simulink model "sinVelToLeader"  (R2016a)
settings: Solver=FixedStepAuto  StartTime=0.0  StopTime=inf  RelTol=1e-3
undefined symbols (not defined in the file or in its folder): Angular, Linear
libraries: robotlib x2
settings Model: Creator=ece446  LastModifiedBy=ece446
settings OptimizationCC: OptimizeModelRefInitCode=on  LifeSpan=Inf  MaxStackSize=64
settings HardwareCC: ProdBitPerPointer=32  ProdLargestAtomicFloat=None  ProdIntDivRoundTo=Undefined  ProdEndianess=Unspecified  ProdWordSize=32  ProdHWDeviceType=Generic->Unspecified (assume 32-bit Generic)  UseEmbeddedCoderFeatures=off
settings RTWCC: SystemTargetFile=ert.tlc  HardwareBoard=Robot Operating System (ROS)  TemplateMakefile=ert_default_tmf  GenerateReport=on  Toolchain=Catkin  IncludeHyperlinkInReport=on  LaunchReport=on  TargetLang=C++  GenerateTraceInfo=on  GenerateTraceReport=on  GenerateTraceReportSl=on  GenerateTraceReportSf=on  GenerateTraceReportEml=on
settings CodeAppCC: ForceParamTrailComments=on  IgnoreCustomStorageClasses=off  OperatorAnnotations=on  SimulinkDataObjDesc=on  SFDataObjDesc=on  MATLABFcnDesc=on  InsertBlockDesc=on  MATLABSourceComments=on
settings ERTTargetCC: SupportNonInlinedSFcns=on

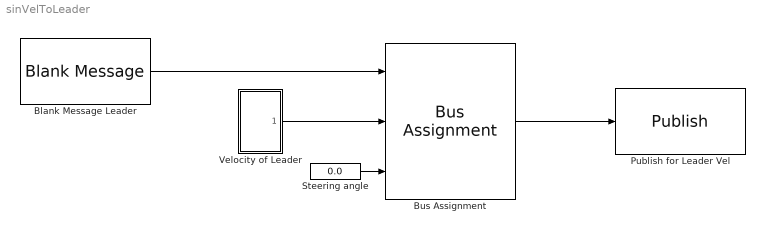
== system sinVelToLeader ==
  Blank Message Leader : robotlib/Blank Message  SourceLibraryInfo=This block requires Robotics System Toolbox  messageType=geometry_msgs/Twist  SampleTime=inf
  Bus Assignment : BusAssignment  AssignedSignals=Linear.X,Angular.Z
  Publish for Leader Vel : robotlib/Publish  SourceLibraryInfo=This block requires Robotics System Toolbox  topicSource=Select from ROS network  topic=/azcar_sim/cmd_vel  messageType=geometry_msgs/Twist  messageQueueLength=1
  Steering angle : Constant  Value=0.0
  Velocity of Leader : Subsystem
  wires:
  Blank Message Leader/1 -> Bus Assignment/1
  Bus Assignment/1 -> Publish for Leader Vel/1
  Velocity of Leader/1(Velocity) -> Bus Assignment/2
  Steering angle/1 -> Bus Assignment/3

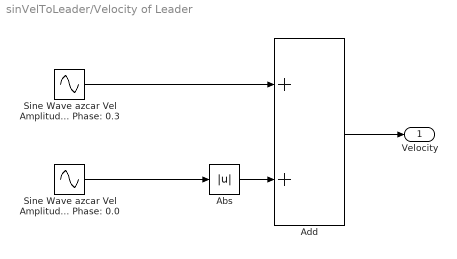
== system sinVelToLeader/Velocity of Leader ==
  Abs : Abs
  Add : Sum
  "Sine Wave azcar Vel Amplitude:5 Frequency: 2 rad/s Phase: 0.3 " : Sin  Amplitude=5  Frequency=2  Phase=0.3  SampleTime=0
  Sine Wave azcar Vel Amplitude:5 Frequency: 3 rad/s Phase: 0.0 : Sin  Amplitude=5  Frequency=3  SampleTime=0
  Velocity : Outport
  wires:
  Sine Wave azcar Vel Amplitude:5 Frequency: 3 rad/s Phase: 0.0/1 -> Abs/1
  Abs/1 -> Add/2
  Add/1 -> Velocity/1
  "Sine Wave azcar Vel Amplitude:5 Frequency: 2 rad/s Phase: 0.3 "/1 -> Add/1
